simulink model "simFxLMS"  (R2018a)
settings: Solver=FixedStepAuto  StartTime=0.0  StopTime=5  FixedStep=1/48000  RelTol=1e-3
values from neighbouring files (symbols this model uses):
  P = P(:)    [run_anc_sim.m]    (also in run_fxlms.m = fir1(80, [60 3000]/(fs/2), 'bandpass'); simWorkSpaceConfig.m = s.w')
  S = load(fullFile)    [fxlms_gui.m]    (also in run_anc_sim.m = S(:); run_fxlms.m = fir1(64, 0.2); simWorkSpaceConfig.m = s.w')
  stepsize = 0.00010    (= 0.0001)    [simWorkSpaceConfig.m]
undefined symbols (not defined in the file or in its folder): magnitude
libraries: simulink x3, dspmathops x3, dspspect3 x3, dspsrcs4 x2, dspstat3 x2
settings Model: Creator=胡子瀚  LastModifiedBy=a
settings DataIOCC: ReturnWorkspaceOutputs=on
settings SFSimCC: SimUseLocalCustomCode=on
settings RTWCC: RTWUseLocalCustomCode=on

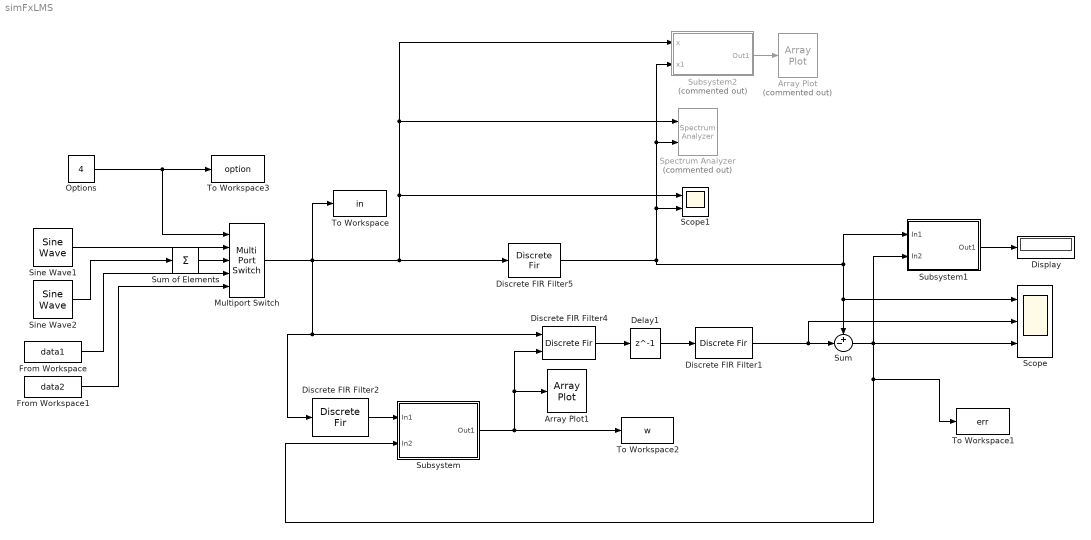
== system simFxLMS ==
  Array Plot : ArrayPlot  Commented=on
  Array Plot1 : ArrayPlot
  Delay1 : Delay  DelayLength=1
  Discrete FIR Filter1 : DiscreteFir  Coefficients=S
  Discrete FIR Filter2 : DiscreteFir  Coefficients=S
  Discrete FIR Filter4 : DiscreteFir  CoefSource=Input port
      settings: InputPortMap=u0,u1
  Discrete FIR Filter5 : DiscreteFir  Coefficients=P
  Display : Display
  From Workspace : FromWorkspace  VariableName=data1  Interpolate=off  OutputAfterFinalValue=Cyclic repetition
  From Workspace1 : FromWorkspace  VariableName=data2  SampleTime=1/48000  Interpolate=off  OutputAfterFinalValue=Cyclic repetition
  Multiport Switch : MultiPortSwitch  Inputs=4
  Options : Constant  Value=4
  Scope : Scope  NumInputPorts=3
  Scope1 : Scope  NumInputPorts=2
  Sine Wave1 : dspsrcs4/Sine Wave  Amplitude=[1]  Frequency=[1000]  Phase=0  SampleMode=Discrete  OutComplex=Real  CompMethod=Trigonometric fcn  TableSize=Speed  SampleTime=1/48000  SamplesPerFrame=1  ResetState=Restart at time zero  OutputFrames=off  dataType=double  wordLen=16  udDataType=sfix(16)  fracBitsMode=Best precision  numFracBits=15  OutDataTypeStr=double  LastOutDataTypeStr=double
  Sine Wave2 : dspsrcs4/Sine Wave  Amplitude=[3 2 1]  Frequency=[310 620 930]  Phase=0  SampleMode=Discrete  OutComplex=Real  CompMethod=Trigonometric fcn  TableSize=Speed  SampleTime=1/48000  SamplesPerFrame=1  ResetState=Restart at time zero  OutputFrames=off  dataType=double  wordLen=16  udDataType=sfix(16)  fracBitsMode=Best precision  numFracBits=15  OutDataTypeStr=double  LastOutDataTypeStr=double
  Spectrum Analyzer : SpectrumAnalyzer  Commented=on  NumInputPorts=2
  Subsystem : Subsystem
  Subsystem1 : Subsystem
  Subsystem2 : Subsystem  Commented=on
  Sum : Sum  Inputs=+-|
  Sum of Elements : Sum  Inputs=+
  To Workspace : ToWorkspace  VariableName=in  SaveFormat=Structure  SampleTime=-1
  To Workspace1 : ToWorkspace  VariableName=err  SaveFormat=Structure  SampleTime=-1
  To Workspace2 : ToWorkspace  VariableName=w  SaveFormat=Structure  SampleTime=-1
  To Workspace3 : ToWorkspace  VariableName=option  SaveFormat=Structure  SampleTime=-1
  wires:
  Discrete FIR Filter1/1 -> Scope/2, Sum/2
  Discrete FIR Filter4/1 -> Delay1/1
  Sine Wave1/1 -> Multiport Switch/2
  Subsystem/1(Out1) -> To Workspace2/1, Array Plot1/1, Discrete FIR Filter4/2
  Delay1/1 -> Discrete FIR Filter1/1
  Discrete FIR Filter5/1 -> Scope/1, Sum/1, Subsystem1/1(In1), Subsystem2/2(x1), Spectrum Analyzer/2, Scope1/2
  Sum/1 -> Subsystem1/2(In2), To Workspace1/1, Subsystem/2(In2), Scope/3
  Subsystem2/1(Out1) -> Array Plot/1
  Subsystem1/1(Out1) -> Display/1
  Multiport Switch/1 -> To Workspace/1, Discrete FIR Filter5/1, Subsystem2/1(x), Spectrum Analyzer/1, Scope1/1, Discrete FIR Filter2/1, Discrete FIR Filter4/1
  Discrete FIR Filter2/1 -> Subsystem/1(In1)
  Sine Wave2/1 -> Sum of Elements/1
  From Workspace/1 -> Multiport Switch/4
  From Workspace1/1 -> Multiport Switch/5
  Sum of Elements/1 -> Multiport Switch/3
  Options/1 -> To Workspace3/1, Multiport Switch/1

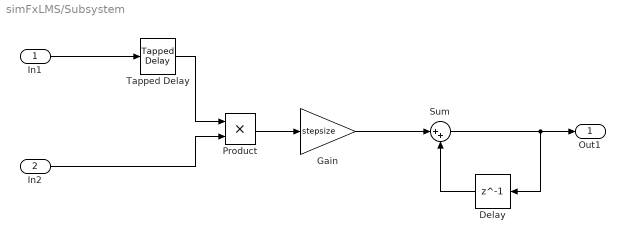
== system simFxLMS/Subsystem ==
  In1 : Inport
  In2 : Inport  Port=2
  Delay : Delay  DelayLength=1
  Gain : Gain  Gain=stepsize
  Product : Product
  Sum : Sum  Inputs=|++
  Tapped Delay : simulink/Discrete/Tapped Delay  vinit=0  samptime=-1  NumDelays=1023  DelayOrder=Newest  includeCurrent=on
  Out1 : Outport  VectorParamsAs1DForOutWhenUnconnected=on
  wires:
  In2/1 -> Product/2
  Product/1 -> Gain/1
  In1/1 -> Tapped Delay/1
  Tapped Delay/1 -> Product/1
  Delay/1 -> Sum/2
  Sum/1 -> Delay/1, Out1/1
  Gain/1 -> Sum/1

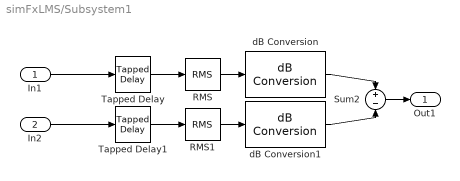
== system simFxLMS/Subsystem1 ==
  In1 : Inport
  In2 : Inport  Port=2
  RMS : dspstat3/RMS  run=off  directionMode=Each column  dimension=1  InputProcessing=Columns as channels (frame based)  reset_popup=None
  RMS1 : dspstat3/RMS  run=off  directionMode=Each column  dimension=1  InputProcessing=Columns as channels (frame based)  reset_popup=None
  Sum2 : Sum  Inputs=+|-
  Tapped Delay : simulink/Discrete/Tapped Delay  vinit=0.0  samptime=-1  NumDelays=20  DelayOrder=Oldest  includeCurrent=off
  Tapped Delay1 : simulink/Discrete/Tapped Delay  vinit=0.0  samptime=-1  NumDelays=20  DelayOrder=Oldest  includeCurrent=off
  dB Conversion : dspmathops/dB Conversion  dBtype=dB  intype=Amplitude  R=1  fuzz=off
      settings: SourceProductName=DSP System Toolbox
  dB Conversion1 : dspmathops/dB Conversion  dBtype=dB  intype=Amplitude  R=1  fuzz=off
      settings: SourceProductName=DSP System Toolbox
  Out1 : Outport  VectorParamsAs1DForOutWhenUnconnected=on
  wires:
  Tapped Delay/1 -> RMS/1
  dB Conversion1/1 -> Sum2/2
  Tapped Delay1/1 -> RMS1/1
  dB Conversion/1 -> Sum2/1
  RMS/1 -> dB Conversion/1
  RMS1/1 -> dB Conversion1/1
  Sum2/1 -> Out1/1
  In1/1 -> Tapped Delay/1
  In2/1 -> Tapped Delay1/1

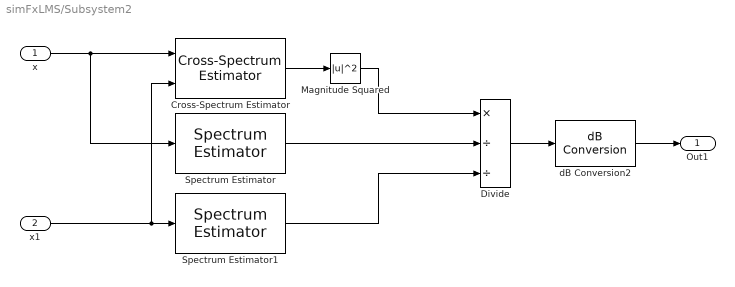
== system simFxLMS/Subsystem2 ==
  x : Inport
  x1 : Inport  Port=2
  Cross-Spectrum Estimator : dspspect3/Cross-Spectrum Estimator  WindowMode=Specify on dialog  WindowLength=1024  Overlap=75  SpectralAverages=1  FFTLengthSource=Auto  FFTLength=128  Window=Hamming  SidelobeAttenuation=60  FrequencyRange=Centered  InheritSampleRate=on  SampleRate=44100  SimulateUsing=Code generation
      settings: SourceProductName=DSP System Toolbox  SourceProductBaseCode=DS
  Divide : Product  Inputs=*//
  Magnitude Squared : Math  Operator=magnitude^2  SaturateOnIntegerOverflow=on
  Spectrum Estimator : dspspect3/Spectrum Estimator  Method=Welch  NumTapsPerBand=1024  SpectrumType=Power  FrequencyResolutionMethod=Window length  FilterBankResolutionMethod=Auto  RBW=5  WindowMode=Specify on dialog  WindowLength=1024  FrequencyBandsSource=Same as input frame size  FrequencyBands=1024  FFTLengthSource=Auto  FFTLength=1024  InheritSampleRate=on  SampleRate=1e-4  Window=Hamming  SidelobeAttenuation=60  SpectralAverages=1  Overlap=75  ReferenceLoad=1  FrequencyRange=Centered  PowerUnits=dBm  OutputMaxHoldSpectrum=off  OutputMinHoldSpectrum=off  OutputFrequencyVector=off  OutputRBW=off  SimulateUsing=Code generation
      settings: SourceProductName=DSP System Toolbox  SourceProductBaseCode=DS
  Spectrum Estimator1 : dspspect3/Spectrum Estimator  Method=Welch  NumTapsPerBand=1024  SpectrumType=Power  FrequencyResolutionMethod=Window length  FilterBankResolutionMethod=Auto  RBW=5  WindowMode=Specify on dialog  WindowLength=1024  FrequencyBandsSource=Same as input frame size  FrequencyBands=1024  FFTLengthSource=Auto  FFTLength=1024  InheritSampleRate=on  SampleRate=1e-4  Window=Hamming  SidelobeAttenuation=60  SpectralAverages=1  Overlap=75  ReferenceLoad=1  FrequencyRange=Centered  PowerUnits=dBm  SimulateUsing=Code generation  OutputMaxHoldSpectrum=off  OutputMinHoldSpectrum=off  OutputFrequencyVector=off  OutputRBW=off
      settings: SourceProductName=DSP System Toolbox  SourceProductBaseCode=DS
  dB Conversion2 : dspmathops/dB Conversion  dBtype=dB  intype=Amplitude  R=1  fuzz=off
      settings: SourceProductName=DSP System Toolbox
  Out1 : Outport  VectorParamsAs1DForOutWhenUnconnected=on
  wires:
  Spectrum Estimator/1 -> Divide/2
  x1/1 -> Cross-Spectrum Estimator/2, Spectrum Estimator1/1
  Spectrum Estimator1/1 -> Divide/3
  Cross-Spectrum Estimator/1 -> Magnitude Squared/1
  x/1 -> Spectrum Estimator/1, Cross-Spectrum Estimator/1
  Magnitude Squared/1 -> Divide/1
  dB Conversion2/1 -> Out1/1
  Divide/1 -> dB Conversion2/1
